simulink model "EST_Simulink"  (R2022a)
settings: Solver=FixedStepAuto  StartTime=0.0  StopTime=T  FixedStep=300  MaxStep=0.05  RelTol=1e-3
values from neighbouring files (symbols this model uses):
  alpha_extraction = 0.1    [EST_Matlab.m]
  alpha_injection = 0.1    [EST_Matlab.m]
  alpha_storage = 0.1    [EST_Matlab.m]
  alpha_transport_from_supply = 0.1    [EST_Matlab.m]
  alpha_transport_to_demand = 0.1    [EST_Matlab.m]
  beta_storage = 1e-8    (= 1e-08)    [EST_Matlab.m]
  E_initial = 0.0*E_storage_max    (= 0)    [EST_Matlab.m]
  E_storage_max = 5e5*MWh    (= 1800000000)    [EST_Matlab.m]
  E_storage_min = 0    [EST_Matlab.m]
settings Model: Creator=joche  LastModifiedBy=20192909
settings DataIOCC: SaveFormat=Array  ReturnWorkspaceOutputs=off

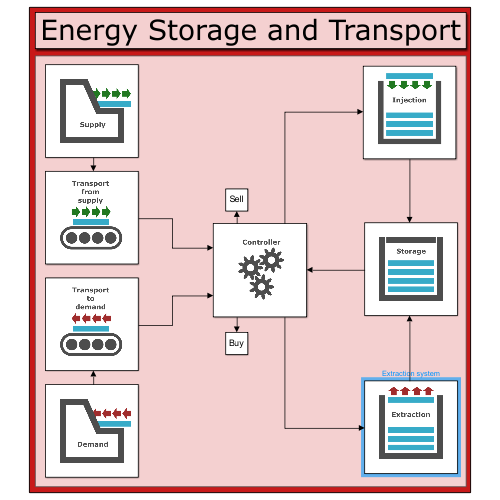
[thumbnail: Simulink's stored preview of the top-level diagram]
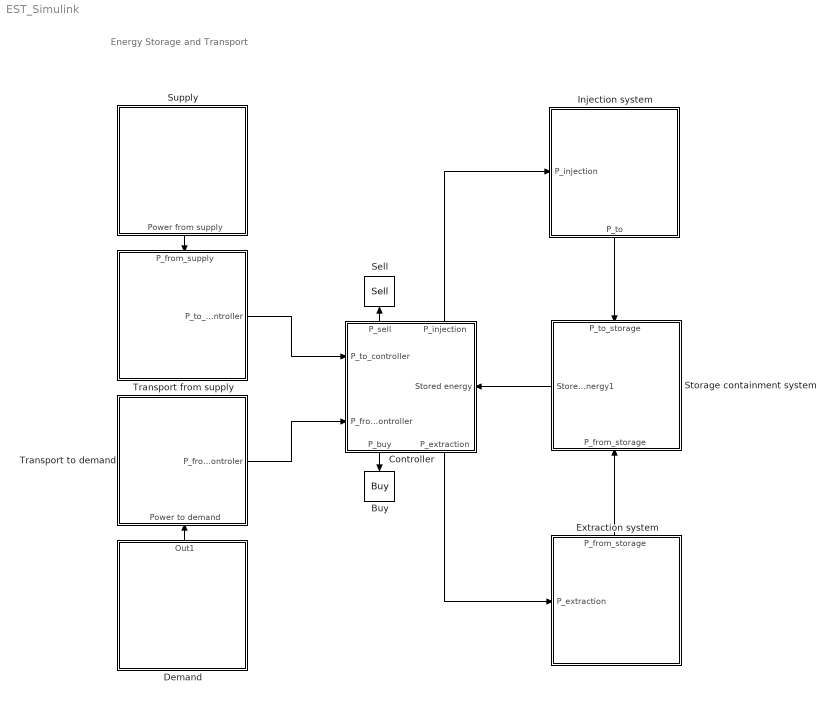
== system EST_Simulink ==
  note: Energy Storage and Transport
  Buy : ToWorkspace  VariableName=Buy  SampleTime=-1
  Controller : Subsystem
      settings: PortSchema="{\"entries\":[{\"content\":{\"sides\":[{\"content\":{\"connectorIds\":[\"In1\",\"In2\"]},\"type\":\"ConnectorPlacement.EquallySpacedRectSide\",\"uuid\":\"4daf33ce-c96a-4783-b5c4-228eed953e01\"},{\"content\":{\"connectorIds\":[\"In3\"],\"side\":\"RIGHT\"},\"type\":\"ConnectorPlacement.EquallySpacedRectSide\",\"uuid\":\"e9942e50-8467-4af8-b79b-80636cbc76e5\"},{\"content\":{\"connectorIds\":[\"Out3\",\"Out4\"],\"side\":\"TOP\"},\"type\":\"ConnectorPlacement.EquallySpacedRectSide\",\"uuid\":\"f315e931-d69b-4751-b712-f89c6c81baeb\"},{\"content\":{\"connectorIds\":[\"Out1\",\"Out2\"],\"side\":\"BOTTOM\"},\"type\":\"ConnectorPlacement.EquallySpacedRectSide\",\"uuid\":\"44715ee6-5cd5-4669-bcb9-5ed7c869bdb3\"}]},\"type\":\"ConnectorPlacement.EquallySpacedConnector\",\"uuid\":\"fff48899-944b-4064-b7d7-ecc12144fb48\"}],\"packageUris\":[\"http://schema.mathworks.com/mf0/Connector/R2020b\"],\"version\":\"1.0\"}"
      mask Display: image('$imagefile'); % Use "Edit Image" on toolstrip to change.
  Demand : Subsystem
      settings: PortSchema="{\"entries\":[{\"content\":{\"sides\":[{\"content\":{},\"type\":\"ConnectorPlacement.EquallySpacedRectSide\",\"uuid\":\"48c6a0df-50e6-4619-b75c-3f0b90ad4772\"},{\"content\":{\"side\":\"RIGHT\"},\"type\":\"ConnectorPlacement.EquallySpacedRectSide\",\"uuid\":\"d0c59a0f-93eb-4811-b50d-4d1a667ea9c0\"},{\"content\":{\"connectorIds\":[\"Out1\"],\"side\":\"TOP\"},\"type\":\"ConnectorPlacement.EquallySpacedRectSide\",\"uuid\":\"b31064d3-46d7-416c-a0ac-4050c2132d29\"}]},\"type\":\"ConnectorPlacement.EquallySpacedConnector\",\"uuid\":\"68b7e5da-bd19-45e6-89e0-e31fb5a00fd0\"}],\"packageUris\":[\"http://schema.mathworks.com/mf0/Connector/R2020b\"],\"version\":\"1.0\"}"
      mask Display: image('$imagefile'); % Use "Edit Image" on toolstrip to change.
  Extraction system : Subsystem
      settings: PortSchema="{\"entries\":[{\"content\":{\"sides\":[{\"content\":{\"connectorIds\":[]},\"type\":\"ConnectorPlacement.EquallySpacedRectSide\",\"uuid\":\"05c5933d-55fc-4e06-853f-fc26d42905f9\"},{\"content\":{\"connectorIds\":[\"In1\"],\"side\":\"RIGHT\"},\"type\":\"ConnectorPlacement.EquallySpacedRectSide\",\"uuid\":\"327426c5-31d5-498b-a2bd-83e49353408c\"},{\"content\":{\"connectorIds\":[],\"side\":\"TOP\"},\"type\":\"ConnectorPlacement.EquallySpacedRectSide\",\"uuid\":\"55306cf3-a3de-4385-a5ae-b8600ecdd5a2\"},{\"content\":{\"connectorIds\":[\"Out1\"],\"side\":\"BOTTOM\"},\"type\":\"ConnectorPlacement.EquallySpacedRectSide\",\"uuid\":\"08fcc9c3-40d3-4ac6-b914-dfeef6039ffb\"}]},\"type\":\"ConnectorPlacement.EquallySpacedConnector\",\"uuid\":\"cb35d5ba-e8c6-462c-b7b2-fe8356d4b0a1\"}],\"packageUris\":[\"http://schema.mathworks.com/mf0/Connector/R2020b\"],\"version\":\"1.0\"}"
      mask Display: image('$imagefile'); % Use "Edit Image" on toolstrip to change.
  Injection system : Subsystem
      settings: PortSchema="{\"entries\":[{\"content\":{\"sides\":[{\"content\":{\"connectorIds\":[]},\"type\":\"ConnectorPlacement.EquallySpacedRectSide\",\"uuid\":\"05c5933d-55fc-4e06-853f-fc26d42905f9\"},{\"content\":{\"connectorIds\":[\"In1\"],\"side\":\"RIGHT\"},\"type\":\"ConnectorPlacement.EquallySpacedRectSide\",\"uuid\":\"327426c5-31d5-498b-a2bd-83e49353408c\"},{\"content\":{\"connectorIds\":[\"Out1\"],\"side\":\"TOP\"},\"type\":\"ConnectorPlacement.EquallySpacedRectSide\",\"uuid\":\"55306cf3-a3de-4385-a5ae-b8600ecdd5a2\"},{\"content\":{\"connectorIds\":[],\"side\":\"BOTTOM\"},\"type\":\"ConnectorPlacement.EquallySpacedRectSide\",\"uuid\":\"08fcc9c3-40d3-4ac6-b914-dfeef6039ffb\"}]},\"type\":\"ConnectorPlacement.EquallySpacedConnector\",\"uuid\":\"cb35d5ba-e8c6-462c-b7b2-fe8356d4b0a1\"}],\"packageUris\":[\"http://schema.mathworks.com/mf0/Connector/R2020b\"],\"version\":\"1.0\"}"
      mask Display: image('$imagefile'); % Use "Edit Image" on toolstrip to change.
  Sell : ToWorkspace  VariableName=Sell  SampleTime=-1
  Storage containment system : Subsystem
      settings: PortSchema="{\"entries\":[{\"content\":{\"sides\":[{\"content\":{\"connectorIds\":[\"Out1\"]},\"type\":\"ConnectorPlacement.EquallySpacedRectSide\",\"uuid\":\"0ba48424-33b9-4934-970f-64fe5d8b070e\"},{\"content\":{\"connectorIds\":[],\"side\":\"RIGHT\"},\"type\":\"ConnectorPlacement.EquallySpacedRectSide\",\"uuid\":\"9cde340f-8f39-4499-9a12-5e1623737660\"},{\"content\":{\"connectorIds\":[\"In1\"],\"side\":\"TOP\"},\"type\":\"ConnectorPlacement.EquallySpacedRectSide\",\"uuid\":\"2af8db04-7fd0-4902-8637-8dc00edb4598\"},{\"content\":{\"connectorIds\":[\"In2\"],\"side\":\"BOTTOM\"},\"type\":\"ConnectorPlacement.EquallySpacedRectSide\",\"uuid\":\"e21ea806-d777-41a3-a53f-556fae66854b\"}]},\"type\":\"ConnectorPlacement.EquallySpacedConnector\",\"uuid\":\"4e2ddb36-4db3-4ab4-858b-ebb8ccefeb1f\"}],\"packageUris\":[\"http://schema.mathworks.com/mf0/Connector/R2020b\"],\"version\":\"1.0\"}"
      mask Display: image('$imagefile'); % Use "Edit Image" on toolstrip to change.
  Supply : Subsystem
      settings: PortSchema="{\"entries\":[{\"content\":{\"sides\":[{\"content\":{\"connectorIds\":[]},\"type\":\"ConnectorPlacement.EquallySpacedRectSide\",\"uuid\":\"48c6a0df-50e6-4619-b75c-3f0b90ad4772\"},{\"content\":{\"connectorIds\":[],\"side\":\"RIGHT\"},\"type\":\"ConnectorPlacement.EquallySpacedRectSide\",\"uuid\":\"d0c59a0f-93eb-4811-b50d-4d1a667ea9c0\"},{\"content\":{\"connectorIds\":[],\"side\":\"TOP\"},\"type\":\"ConnectorPlacement.EquallySpacedRectSide\",\"uuid\":\"b31064d3-46d7-416c-a0ac-4050c2132d29\"},{\"content\":{\"connectorIds\":[\"Out1\"],\"side\":\"BOTTOM\"},\"type\":\"ConnectorPlacement.EquallySpacedRectSide\",\"uuid\":\"efd38a8d-1399-4a01-964d-0e5be53ae090\"}]},\"type\":\"ConnectorPlacement.EquallySpacedConnector\",\"uuid\":\"68b7e5da-bd19-45e6-89e0-e31fb5a00fd0\"}],\"packageUris\":[\"http://schema.mathworks.com/mf0/Connector/R2020b\"],\"version\":\"1.0\"}"
      mask Display: image('$imagefile'); % Use "Edit Image" on toolstrip to change.
  Transport from supply : Subsystem
      settings: PortSchema="{\"entries\":[{\"content\":{\"sides\":[{\"content\":{\"connectorIds\":[]},\"type\":\"ConnectorPlacement.EquallySpacedRectSide\",\"uuid\":\"31329006-3d36-4d93-9c44-7503a515d397\"},{\"content\":{\"connectorIds\":[\"Out1\"],\"side\":\"RIGHT\"},\"type\":\"ConnectorPlacement.EquallySpacedRectSide\",\"uuid\":\"aba139c7-f9b6-4881-a56b-a4cbbedacd88\"},{\"content\":{\"connectorIds\":[\"In1\"],\"side\":\"TOP\"},\"type\":\"ConnectorPlacement.EquallySpacedRectSide\",\"uuid\":\"e683eb73-7a35-4160-9c39-da83856a6278\"}]},\"type\":\"ConnectorPlacement.EquallySpacedConnector\",\"uuid\":\"804af608-1d70-444f-af69-e05f19bf98f3\"}],\"packageUris\":[\"http://schema.mathworks.com/mf0/Connector/R2020b\"],\"version\":\"1.0\"}"
      mask Display: image('$imagefile'); % Use "Edit Image" on toolstrip to change.
  Transport to demand : Subsystem
      settings: PortSchema="{\"entries\":[{\"content\":{\"sides\":[{\"content\":{\"connectorIds\":[]},\"type\":\"ConnectorPlacement.EquallySpacedRectSide\",\"uuid\":\"31329006-3d36-4d93-9c44-7503a515d397\"},{\"content\":{\"connectorIds\":[\"Out1\"],\"side\":\"RIGHT\"},\"type\":\"ConnectorPlacement.EquallySpacedRectSide\",\"uuid\":\"aba139c7-f9b6-4881-a56b-a4cbbedacd88\"},{\"content\":{\"connectorIds\":[],\"side\":\"TOP\"},\"type\":\"ConnectorPlacement.EquallySpacedRectSide\",\"uuid\":\"e683eb73-7a35-4160-9c39-da83856a6278\"},{\"content\":{\"connectorIds\":[\"In1\"],\"side\":\"BOTTOM\"},\"type\":\"ConnectorPlacement.EquallySpacedRectSide\",\"uuid\":\"c378138f-7233-4483-870c-40a69b3495ee\"}]},\"type\":\"ConnectorPlacement.EquallySpacedConnector\",\"uuid\":\"804af608-1d70-444f-af69-e05f19bf98f3\"}],\"packageUris\":[\"http://schema.mathworks.com/mf0/Connector/R2020b\"],\"version\":\"1.0\"}"
      mask Display: image('$imagefile'); % Use "Edit Image" on toolstrip to change.
  wires:
  Supply/1(Power from supply) -> Transport from supply/1(P_from_supply)
  Transport from supply/1(P_to_controller) -> Controller/1(P_to_controller)
  Transport to demand/1(P_from_controler) -> Controller/2(P_from_controller)
  Demand/1(Out1) -> Transport to demand/1(Power to demand)
  Controller/3(P_sell) -> Sell/1
  Controller/1(P_buy) -> Buy/1
  Controller/2(P_extraction) -> Extraction system/1(P_extraction)
  Injection system/1(P_to) -> Storage containment system/1(P_to_storage)
  Extraction system/1(P_from_storage) -> Storage containment system/2(P_from_storage)
  Storage containment system/1(Stored energy1) -> Controller/3(Stored energy)
  Controller/4(P_injection) -> Injection system/1(P_injection)

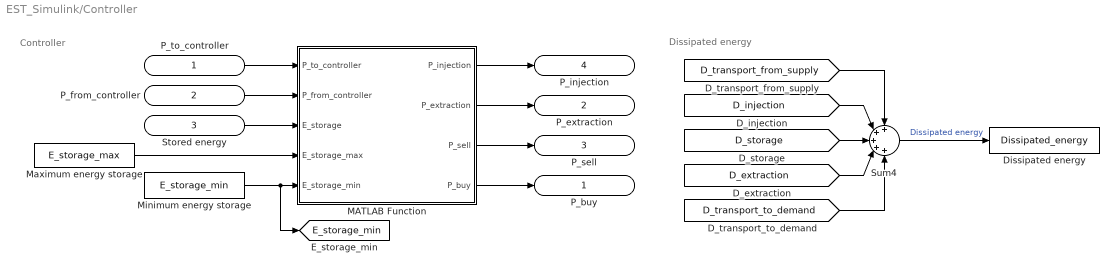
== system EST_Simulink/Controller ==
  note: Dissipated energy
  note: Controller
  P_to_controller : Inport
  P_from_controller : Inport  Port=2
  Stored energy : Inport  Port=3
  Dissipated energy : ToWorkspace  VariableName=Dissipated_energy  SampleTime=-1
  MATLAB Function : MATLAB Function  TreatAsAtomicUnit=on
  Maximum energy storage : Constant  Value=E_storage_max
  Minimum energy storage : Constant  Value=E_storage_min
  Sum4 : Sum  Inputs=+++++
  P_buy : Outport
  P_extraction : Outport  Port=2
  P_sell : Outport  Port=3
  P_injection : Outport  Port=4
  tag scope: E_storage_min=global
  wires:
  P_from_controller/1 -> MATLAB Function/2(P_from_controller)
  MATLAB Function/2(P_extraction) -> P_extraction/1
  MATLAB Function/3(P_sell) -> P_sell/1
  MATLAB Function/4(P_buy) -> P_buy/1
  Minimum energy storage/1 -> [E_storage_min], MATLAB Function/5(E_storage_min)
  Maximum energy storage/1 -> MATLAB Function/4(E_storage_max)
  P_to_controller/1 -> MATLAB Function/1(P_to_controller)
  MATLAB Function/1(P_injection) -> P_injection/1
  Stored energy/1 -> MATLAB Function/3(E_storage)
  [D_extraction] -> Sum4/4
  [D_transport_to_demand] -> Sum4/5
  Sum4/1 -> Dissipated energy/1  "Dissipated energy"
  [D_transport_from_supply] -> Sum4/1
  [D_injection] -> Sum4/2
  [D_storage] -> Sum4/3

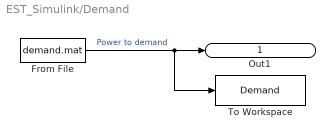
== system EST_Simulink/Demand ==
  From File : FromFile  FileName=demand.mat  SampleTime=0
  To Workspace : ToWorkspace  VariableName=Demand  SampleTime=-1
  Out1 : Outport
  wires:
  From File/1 -> To Workspace/1, Out1/1  "Power to demand"

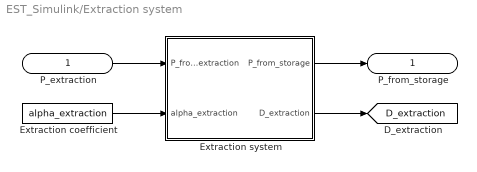
== system EST_Simulink/Extraction system ==
  P_extraction : Inport
  Extraction coefficient : Constant  Value=alpha_extraction
  Extraction system : MATLAB Function  TreatAsAtomicUnit=on
  P_from_storage : Outport
  tag scope: D_extraction=global
  wires:
  P_extraction/1 -> Extraction system/1(P_from_extraction)
  Extraction system/1(P_from_storage) -> P_from_storage/1
  Extraction coefficient/1 -> Extraction system/2(alpha_extraction)
  Extraction system/2(D_extraction) -> [D_extraction]

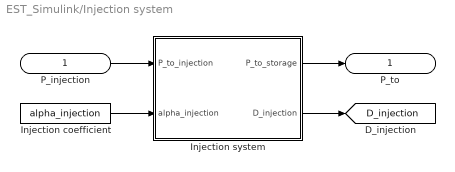
== system EST_Simulink/Injection system ==
  P_injection : Inport
  Injection coefficient : Constant  Value=alpha_injection
  Injection system : MATLAB Function  TreatAsAtomicUnit=on
  P_to : Outport
  tag scope: D_injection=global
  wires:
  P_injection/1 -> Injection system/1(P_to_injection)
  Injection system/1(P_to_storage) -> P_to/1
  Injection coefficient/1 -> Injection system/2(alpha_injection)
  Injection system/2(D_injection) -> [D_injection]

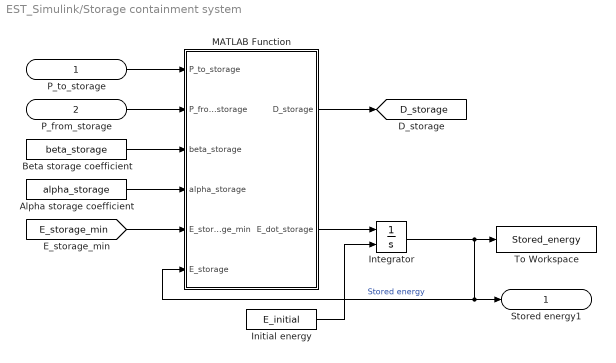
== system EST_Simulink/Storage containment system ==
  P_to_storage : Inport
  P_from_storage : Inport  Port=2
  Alpha storage coefficient : Constant  Value=alpha_storage
  Beta storage coefficient : Constant  Value=beta_storage
  Initial energy : Constant  Value=E_initial
  Integrator : Integrator  InitialConditionSource=external
  MATLAB Function : MATLAB Function  TreatAsAtomicUnit=on
  To Workspace : ToWorkspace  VariableName=Stored_energy  SampleTime=-1
  Stored energy1 : Outport
  tag scope: D_storage=global
  wires:
  P_from_storage/1 -> MATLAB Function/2(P_from_storage)
  P_to_storage/1 -> MATLAB Function/1(P_to_storage)
  Initial energy/1 -> Integrator/2
  Integrator/1 -> MATLAB Function/6(E_storage), Stored energy1/1, To Workspace/1  "Stored energy"
  MATLAB Function/1(D_storage) -> [D_storage]
  Beta storage coefficient/1 -> MATLAB Function/3(beta_storage)
  MATLAB Function/2(E_dot_storage) -> Integrator/1
  [E_storage_min] -> MATLAB Function/5(E_storage_min)
  Alpha storage coefficient/1 -> MATLAB Function/4(alpha_storage)

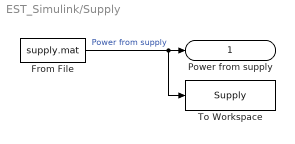
== system EST_Simulink/Supply ==
  From File : FromFile  FileName=supply.mat  SampleTime=0
  To Workspace : ToWorkspace  VariableName=Supply  SampleTime=-1
  Power from supply : Outport
  wires:
  From File/1 -> To Workspace/1, Power from supply/1  "Power from supply"

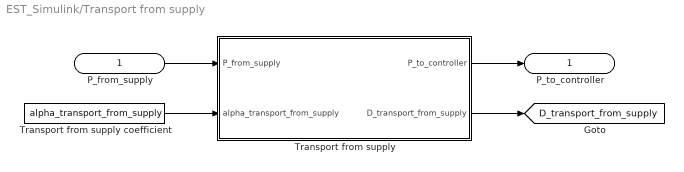
== system EST_Simulink/Transport from supply ==
  P_from_supply : Inport
  Transport from supply : MATLAB Function  TreatAsAtomicUnit=on
  Transport from supply coefficient : Constant  Value=alpha_transport_from_supply
  P_to_controller : Outport
  tag scope: D_transport_from_supply=global
  wires:
  Transport from supply coefficient/1 -> Transport from supply/2(alpha_transport_from_supply)
  P_from_supply/1 -> Transport from supply/1(P_from_supply)
  Transport from supply/1(P_to_controller) -> P_to_controller/1
  Transport from supply/2(D_transport_from_supply) -> [D_transport_from_supply]

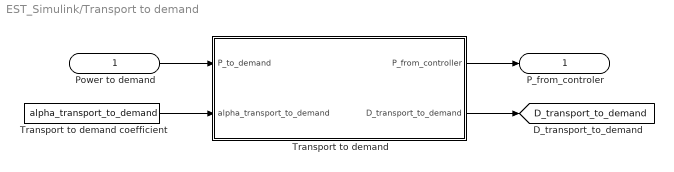
== system EST_Simulink/Transport to demand ==
  Power to demand : Inport
  Transport to demand : MATLAB Function  TreatAsAtomicUnit=on
  Transport to demand coefficient : Constant  Value=alpha_transport_to_demand
  P_from_controler : Outport
  tag scope: D_transport_to_demand=global
  wires:
  Transport to demand coefficient/1 -> Transport to demand/2(alpha_transport_to_demand)
  Power to demand/1 -> Transport to demand/1(P_to_demand)
  Transport to demand/1(P_from_controller) -> P_from_controler/1
  Transport to demand/2(D_transport_to_demand) -> [D_transport_to_demand]

== matlab function EST_Simulink/Injection system/Injection system ==
  data: P_to_injection input; P_to_storage output; alpha_injection input; D_injection output
function [P_to_storage, D_injection] = injection(P_to_injection, alpha_injection)
    D_injection = alpha_injection * P_to_injection;
    P_to_storage = P_to_injection - D_injection;

== matlab function EST_Simulink/Transport from supply/Transport from supply ==
  data: P_from_supply input; P_to_controller output; alpha_transport_from_supply input; D_transport_from_supply output
function [P_to_controller, D_transport_from_supply] = transport_from_supply(P_from_supply, alpha_transport_from_supply)
    D_transport_from_supply = alpha_transport_from_supply * P_from_supply;
    P_to_controller = P_from_supply - D_transport_from_supply;

== matlab function EST_Simulink/Controller/MATLAB Function ==
  data: P_injection output; P_extraction output; P_sell output; P_buy output; P_to_controller input; P_from_controller input; E_storage input; E_storage_max input; E_storage_min input
function [P_injection, P_extraction, P_sell, P_buy] = controller(P_to_controller, P_from_controller, E_storage, E_storage_max, E_storage_min)

    %%%%%%%%%%%%%%%%%%%%%%%%%%%%%
    % Power surplus or deficit %
    %%%%%%%%%%%%%%%%%%%%%%%%%%%%%

    Delta_P = P_to_controller - P_from_controller;

    % Power surplus
    if Delta_P >= 0

        %%%%%%%%%%%%%%%%%%%%%
        % Storage injection %
        %%%%%%%%%%%%%%%%%%%%%

        % Storage system is not full
        if E_storage < E_storage_max 

            P_injection = Delta_P;

        % Storage system is full
        else
            P_injection = 0;
        end

        %%%%%%%%%%%%%%%%%%%%%%
        % Storage extraction %
        %%%%%%%%%%%%%%%%%%%%%%

        P_extraction = 0;

        %%%%%%%%%%%%%%%%%%%%%
        % Load-balancing    %
        %%%%%%%%%%%%%%%%%%%%%

        P_sell = Delta_P - P_injection;
        P_buy  = 0;

    % Power deficit
    else
        %%%%%%%%%%%%%%%%%%%%%
        % Storage injection %
        %%%%%%%%%%%%%%%%%%%%%

        P_injection = 0;

        %%%%%%%%%%%%%%%%%%%%%%
        % Storage extraction %
        %%%%%%%%%%%%%%%%%%%%%%

        % Storage system is not empty
        if E_storage > E_storage_min

            P_extraction = -Delta_P;

        % Storage system is empty
        else
            P_extraction = 0;
        end

        %%%%%%%%%%%%%%%%%%%%%
        % Load-balancing    %
        %%%%%%%%%%%%%%%%%%%%%

        P_sell = 0;
        P_buy  = -Delta_P - P_extraction;
    end

== matlab function EST_Simulink/Extraction system/Extraction system ==
  data: P_from_extraction input; P_from_storage output; alpha_extraction input; D_extraction output
function [P_from_storage, D_extraction] = extraction(P_from_extraction, alpha_extraction)
    D_extraction = alpha_extraction / (1-alpha_extraction) * P_from_extraction;
    P_from_storage = P_from_extraction + D_extraction;

== matlab function EST_Simulink/Storage containment system/MATLAB Function ==
  data: D_storage output; E_dot_storage output; P_to_storage input; P_from_storage input; beta_storage input; alpha_storage input; E_storage_min input; E_storage input
function [D_storage, E_dot_storage]= Storage(P_to_storage, P_from_storage, beta_storage, alpha_storage , E_storage_min, E_storage)
    D_storage = 1 / (1+alpha_storage) * beta_storage * (E_storage-E_storage_min) + alpha_storage / (1+alpha_storage) * (P_to_storage-P_from_storage);
    E_dot_storage = P_to_storage - P_from_storage-D_storage;

== matlab function EST_Simulink/Transport to demand/Transport to demand ==
  data: P_to_demand input; P_from_controller output; alpha_transport_to_demand input; D_transport_to_demand output
function [P_from_controller, D_transport_to_demand] = transport_to_demand(P_to_demand, alpha_transport_to_demand)
    D_transport_to_demand = alpha_transport_to_demand / (1-alpha_transport_to_demand) * P_to_demand;
    P_from_controller = P_to_demand + D_transport_to_demand;
